simulink model "PID_Controller"  (R2020a)
settings: Solver=VariableStepAuto  StartTime=0.0  StopTime=120  RelTol=1e-3
values from neighbouring files (symbols this model uses):
  kd = 40    [w2p3.mat]
  ki = 40    [w2p3.mat]
  kp = 800    [w2p3.mat]
settings Model: Creator=Shubham  LastModifiedBy=Shubham
settings DataIOCC: SaveOutput=off  SaveTime=off

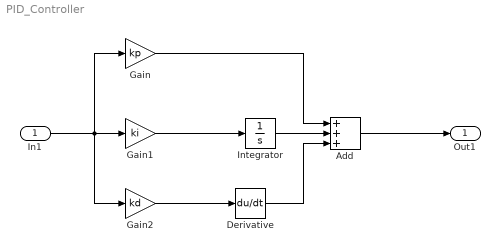
== system PID_Controller ==
  In1 : Inport  OutDataTypeStr=double  PortDimensions=1  SampleTime=0
  Add : Sum  Inputs=+++
  Derivative : Derivative
  Gain : Gain  Gain=kp
  Gain1 : Gain  Gain=ki
  Gain2 : Gain  Gain=kd
  Integrator : Integrator
  Out1 : Outport  OutDataTypeStr=double  PortDimensions=1  SampleTime=0
  wires:
  Gain1/1 -> Integrator/1
  In1/1 -> Gain1/1, Gain/1, Gain2/1
  Integrator/1 -> Add/2
  Add/1 -> Out1/1
  Gain2/1 -> Derivative/1
  Gain/1 -> Add/1
  Derivative/1 -> Add/3
